simulink model "HYV_EMR_IBC_Macro_2022a"  (R2022a)
settings: Solver=ode45  StartTime=SIM.t_min  StopTime=SIM.t_simul  FixedStep=1e-2  MaxStep=10e-3  RelTol=1e-3  EnableMultiTasking=on
InitFcn:
  | init_hyv
undefined symbols (not defined in the file or in its folder): BATp, CHAp, CYCL, EDp, EMp, ICE, MTp, Paux, RDp, REDR, RegV
libraries: simulink x2
settings Model: ExtModeTrigMode=oneshot  ExtModeArmWhenConnect=off  Creator=Tony  LastModifiedBy=philippe.barrade
settings SolverCC: ZeroCrossAlgorithm=Non-adaptive  AlgebraicLoopSolver=TrustRegion
settings DataIOCC: SaveFormat=Array  SignalLoggingSaveFormat=ModelDataLogs  ReturnWorkspaceOutputs=off  SignalLoggingName=sigsOut
settings OptimizationCC: BooleanDataType=off  ExpressionDepthLimit=2147483647  LifeSpan=inf
settings DebuggingCC: SaveWithParameterizedLinksMsg=none  UnderspecifiedInitializationDetection=Classic  MergeDetectMultiDrivingBlocksExec=none  SignalResolutionControl=TryResolveAllWithWarning  MultiTaskDSMMsg=warning  MultiTaskCondExecSysMsg=none  FcnCallInpInsideContextMsg=warning  UnconnectedInputMsg=warning  UnconnectedOutputMsg=warning  UnconnectedLineMsg=warning  StateNameClashWarn=warning  SFUnexpectedBacktrackingDiag=warning  SFNoUnconditionalDefaultTransitionDiag=warning  ArithmeticOperatorsInVariantConditions=warning
settings HardwareCC: ProdBitPerPointer=32  ProdBitPerSizeT=32  ProdBitPerPtrDiffT=32  ProdLargestAtomicFloat=None  ProdIntDivRoundTo=Undefined  ProdEndianess=Unspecified  ProdWordSize=32  ProdHWDeviceType=32-bit Generic  TargetUnknown=on
settings ModelReferenceCC: PropagateSignalLabelsOutOfModel=off
settings SFSimCC: CustomCodeUndefinedFunction=UseInterfaceOnly
settings CodeAppCC: StateflowObjectComments=on
settings GRTTargetCC: TargetLangStandard=C89/C90 (ANSI)  CombineOutputUpdateFcns=off  GRTInterface=on
settings ConfigComp: CovMetricSettings=dw  CovSaveCumulativeToWorkspaceVar=on  CovSaveSingleToWorkspaceVar=on

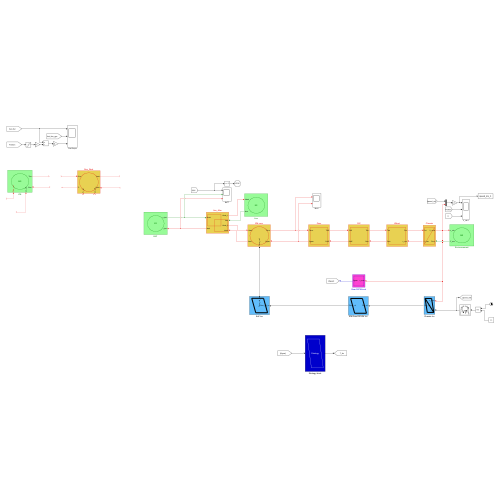
[thumbnail: Simulink's stored preview of the top-level diagram]
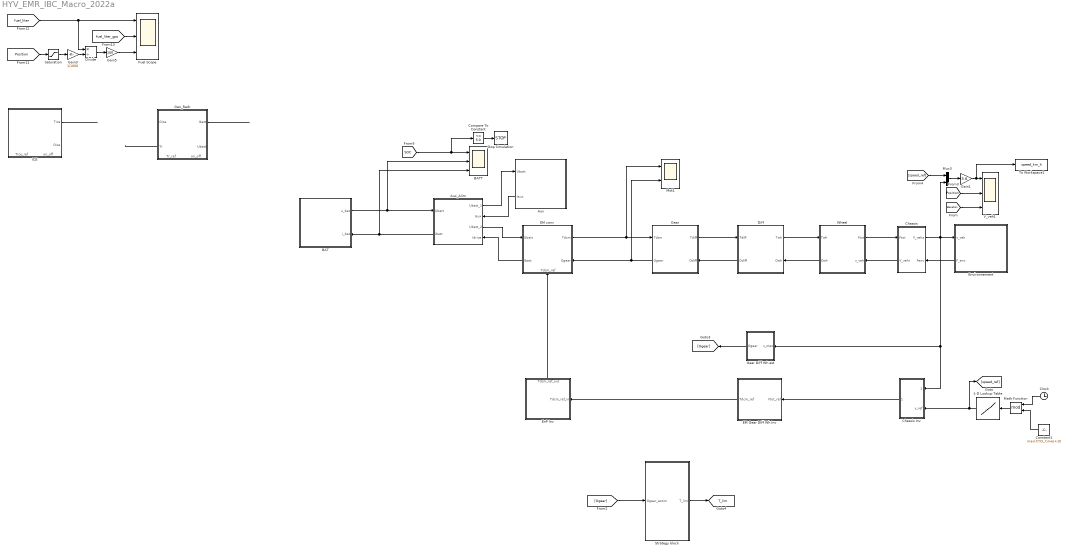
== system HYV_EMR_IBC_Macro_2022a ==
  1-D Lookup Table : Lookup_n-D  NumberOfTableDimensions=1  BreakpointsForDimension1=CYCL.time  Table=CYCL.speed  InternalRulePriority=Speed  RndMeth=Simplest
  Aux : Subsystem
      settings: PortSchema="{\"entries\":[{\"content\":{\"sides\":[{\"content\":{\"connectorIds\":[\"In1\",\"Out1\"]},\"type\":\"ConnectorPlacement.EquallySpacedRectSide\",\"uuid\":\"e57ce769-5dfa-4323-9199-18ff4bf0cf0d\"},{\"content\":{\"side\":\"RIGHT\"},\"type\":\"ConnectorPlacement.EquallySpacedRectSide\",\"uuid\":\"ab409fab-d314-4206-bddf-ed026c86ef76\"},{\"content\":{\"side\":\"TOP\"},\"type\":\"ConnectorPlacement.EquallySpacedRectSide\",\"uuid\":\"b908e240-8ad5-4078-8f5b-5b2bce20148c\"}]},\"type\":\"ConnectorPlacement.EquallySpacedConnector\",\"uuid\":\"97ae4631-eb25-4761-beab-92c01239a3fc\"}],\"packageUris\":[\"http://schema.mathworks.com/mf0/Connector/R2020b\"],\"version\":\"1.0\"}"
      mask Display:
      | plot(0,0,100,100, 1.2*[50,57.68,60.77,63.08,64.97,66.58,68,69.26,70.4, 	71.42,72.36,78.28,80,78.28,72.36,71.42,70.4, 	69.26,68,66.58,64.97,63.08,60.77,57.68,50,42.32, 	39.23,36.92,35.03,33.42,32,30.74,29.6,28.58, 	27.64,21.72,20,21.72,27.64,28.58,29.6,30.74,32, 	33.42,35.03,36.92,39.23,42.32,50]-10, 1.2*[20,21,22,23,24,25,26,27,28,29,30,40,50,60,70,71,72, 	73,74,75,76,77,78,79,80,79,78,77,76,75,74,73,72, 	71,70,60,50,40,30,29,28,27,26,25,24,23,22,21,20]-10)
      | disp('ES')
  Aux_Alim : Subsystem  mask(CM){}
      settings: PortSchema="{\"entries\":[{\"content\":{\"sides\":[{\"content\":{\"connectorIds\":[\"In1\",\"Out3\"]},\"type\":\"ConnectorPlacement.EquallySpacedRectSide\",\"uuid\":\"fe3b80e5-6bea-4454-b396-78d68e4e0983\"},{\"content\":{\"connectorIds\":[\"Out1\",\"In2\",\"Out2\",\"In3\"],\"side\":\"RIGHT\"},\"type\":\"ConnectorPlacement.EquallySpacedRectSide\",\"uuid\":\"fd9b9ae6-7a3e-4ad6-b5ff-7ff0e231c6c1\"},{\"content\":{\"side\":\"TOP\"},\"type\":\"ConnectorPlacement.EquallySpacedRectSide\",\"uuid\":\"d806e031-cf18-4ebb-a7e2-aa884fb49c19\"}]},\"type\":\"ConnectorPlacement.EquallySpacedConnector\",\"uuid\":\"fbb11b08-f3d2-4dd1-a8d6-045eff655811\"}],\"packageUris\":[\"http://schema.mathworks.com/mf0/Connector/R2020b\"],\"version\":\"1.0\"}"
      mask Display: plot(0,0,100,100,[35,35,95,95,35],[65,10,10,65,65], [5,5,65,65,5],[90,35,35,90,90])
  BAT : Subsystem
      settings: PortSchema="{\"entries\":[{\"content\":{\"sides\":[{\"content\":{\"connectorIds\":[]},\"type\":\"ConnectorPlacement.EquallySpacedRectSide\",\"uuid\":\"f966fbbf-87fd-4eae-ac75-d366ea856ba9\"},{\"content\":{\"connectorIds\":[\"Out1\",\"In1\"],\"side\":\"RIGHT\"},\"type\":\"ConnectorPlacement.EquallySpacedRectSide\",\"uuid\":\"019a522f-a65b-4de4-928a-6ec503aa07e1\"},{\"content\":{\"connectorIds\":[],\"side\":\"TOP\"},\"type\":\"ConnectorPlacement.EquallySpacedRectSide\",\"uuid\":\"2e7350c2-17d6-436e-acd0-d7bc7ebcdc21\"}]},\"type\":\"ConnectorPlacement.EquallySpacedConnector\",\"uuid\":\"cf36ffa8-c853-4b91-8b40-e4ddcf06bdb1\"}],\"packageUris\":[\"http://schema.mathworks.com/mf0/Connector/R2020b\"],\"version\":\"1.0\"}"
      mask Display:
      | plot(0,0,100,100, 1.2*[50,57.68,60.77,63.08,64.97,66.58,68,69.26,70.4, 	71.42,72.36,78.28,80,78.28,72.36,71.42,70.4, 	69.26,68,66.58,64.97,63.08,60.77,57.68,50,42.32, 	39.23,36.92,35.03,33.42,32,30.74,29.6,28.58, 	27.64,21.72,20,21.72,27.64,28.58,29.6,30.74,32, 	33.42,35.03,36.92,39.23,42.32,50]-10, 1.2*[20,21,22,23,24,25,26,27,28,29,30,40,50,60,70,71,72, 	73,74,75,76,77,78,79,80,79,78,77,76,75,74,73,72, 	71,70,60,50,40,30,29,28,27,26,25,24,23,22,21,20]-10)
      | disp('ES')
  BATT : Scope  NumInputPorts=3
  Chassis : Subsystem  mask(CM){}
      settings: PortSchema="{\"entries\":[{\"content\":{\"sides\":[{\"content\":{\"connectorIds\":[\"In1\",\"Out2\"]},\"type\":\"ConnectorPlacement.EquallySpacedRectSide\",\"uuid\":\"620ffb90-6f06-474c-af56-4865758ad724\"},{\"content\":{\"connectorIds\":[\"Out1\",\"In2\"],\"side\":\"RIGHT\"},\"type\":\"ConnectorPlacement.EquallySpacedRectSide\",\"uuid\":\"7a4bba18-9bee-4c5d-b60c-6ae6fbfa3157\"},{\"content\":{\"connectorIds\":[],\"side\":\"TOP\"},\"type\":\"ConnectorPlacement.EquallySpacedRectSide\",\"uuid\":\"2f500b5d-e16a-4b09-8380-9fc4853d3c00\"}]},\"type\":\"ConnectorPlacement.EquallySpacedConnector\",\"uuid\":\"25a91873-aa5a-4f00-84d2-bf925e985f7d\"}],\"packageUris\":[\"http://schema.mathworks.com/mf0/Connector/R2020b\"],\"version\":\"1.0\"}"
      mask Display: plot(0,0,100,100,[10,10,90,90,10],[90,10,10,90,90], [10,90],[10,90])
  Chassis Inv : Subsystem
      mask Display: plot(0,0,100,100, [10,30,90,70,10,90],[90,10,10,90,90,10])
  Clock : Clock
  Compare To Constant : simulink/Logic and Bit Operations/Compare To Constant  relop=<=  const=5.0  OutDataTypeStr=boolean
  Constant1 : Constant  Value=max(CYCL.time)+10
  Diff : Subsystem  mask(Hacheur){}
      settings: PortSchema="{\"entries\":[{\"content\":{\"sides\":[{\"content\":{\"connectorIds\":[\"In1\",\"Out2\"]},\"type\":\"ConnectorPlacement.EquallySpacedRectSide\",\"uuid\":\"61fbc010-38ff-4a80-98f4-f5d8a9e77fd8\"},{\"content\":{\"connectorIds\":[\"Out1\",\"In2\"],\"side\":\"RIGHT\"},\"type\":\"ConnectorPlacement.EquallySpacedRectSide\",\"uuid\":\"7ae9e15d-ee0f-4ba6-b3b7-5dcbca441e0a\"},{\"content\":{\"connectorIds\":[],\"side\":\"TOP\"},\"type\":\"ConnectorPlacement.EquallySpacedRectSide\",\"uuid\":\"f4fbe656-3ef3-486e-b25e-f340040f3905\"},{\"content\":{\"connectorIds\":[],\"side\":\"BOTTOM\"},\"type\":\"ConnectorPlacement.EquallySpacedRectSide\",\"uuid\":\"e8cc994c-4958-42b4-b139-c82ce4c5ea4a\"}]},\"type\":\"ConnectorPlacement.EquallySpacedConnector\",\"uuid\":\"024d92c1-e2c4-4b69-9482-c403c9d240aa\"}],\"packageUris\":[\"http://schema.mathworks.com/mf0/Connector/R2020b\"],\"version\":\"1.0\"}"
      mask Display: plot(0,0,100,100,[10,10,90,90,10],[90,10,10,90,90])
  Divide : Product  Inputs=*/
  EM Gear DIff Wh Inv : Subsystem
      mask Display: plot(0,0,100,100,[10,30,90,70,10],[90,10,10,90,90])
  EM conv : Subsystem
      settings: PortSchema="{\"entries\":[{\"content\":{\"sides\":[{\"content\":{\"connectorIds\":[\"In1\",\"Out2\"]},\"type\":\"ConnectorPlacement.EquallySpacedRectSide\",\"uuid\":\"aa766bd2-1e00-44a9-a500-41c2a98848e3\"},{\"content\":{\"connectorIds\":[\"Out1\",\"In3\"],\"side\":\"RIGHT\"},\"type\":\"ConnectorPlacement.EquallySpacedRectSide\",\"uuid\":\"49bb6889-ad6c-456e-94dd-aff29c8ca84c\"},{\"content\":{\"side\":\"TOP\"},\"type\":\"ConnectorPlacement.EquallySpacedRectSide\",\"uuid\":\"33b42b41-d96e-4f45-af15-b9a879923102\"},{\"content\":{\"connectorIds\":[\"In2\"],\"side\":\"BOTTOM\"},\"type\":\"ConnectorPlacement.EquallySpacedRectSide\",\"uuid\":\"830b03b5-14ae-4cee-8c80-baeec75b28b0\"}]},\"type\":\"ConnectorPlacement.EquallySpacedConnector\",\"uuid\":\"59a0cd24-e9fa-4621-b3e9-3869a068d1ef\"}],\"packageUris\":[\"http://schema.mathworks.com/mf0/Connector/R2020b\"],\"version\":\"1.0\"}"
      mask Display: plot(0,0,100,100, 1.4*[50,57.68,60.77,63.08,64.97,66.58,68,69.26,70.4, 	71.42,72.36,78.28,80,78.28,72.36,71.42,70.4, 	69.26,68,66.58,64.97,63.08,60.77,57.68,50,42.32, 	39.23,36.92,35.03,33.42,32,30.74,29.6,28.58, 	27.64,21.72,20,21.72,27.64,28.58,29.6,30.74,32, 	33.42,35.03,36.92,39.23,42.32,50]-20, 1.4*[20,21,22,23,24,25,26,27,28,29,30,40,50,60,70,71,72, 	73,74,75,76,77,78,79,80,79,78,77,76,75,74,73,72, 	71,70,60,50,40,30,29,28,27,26,25,24,23,22,21,20]-20)
  EnP Inv : Subsystem
      settings: PortSchema="{\"entries\":[{\"content\":{\"sides\":[{\"content\":{\"connectorIds\":[\"In1\"]},\"type\":\"ConnectorPlacement.EquallySpacedRectSide\",\"uuid\":\"39dcb6ca-7d3c-49e9-8aff-6e45c752a7e4\"},{\"content\":{\"side\":\"RIGHT\"},\"type\":\"ConnectorPlacement.EquallySpacedRectSide\",\"uuid\":\"f02eeddd-07d1-428e-b420-27aa15bc8886\"},{\"content\":{\"connectorIds\":[\"Out1\"],\"side\":\"TOP\"},\"type\":\"ConnectorPlacement.EquallySpacedRectSide\",\"uuid\":\"752f1347-9d6b-4136-bea0-6d91d7e60b0a\"}]},\"type\":\"ConnectorPlacement.EquallySpacedConnector\",\"uuid\":\"f213fa59-4ba1-490d-8e30-b1e1c9b24a7e\"}],\"packageUris\":[\"http://schema.mathworks.com/mf0/Connector/R2020b\"],\"version\":\"1.0\"}"
      mask Display: plot(0,0,100,100,[10,30,90,70,10],[90,10,10,90,90])
  Environnement : Subsystem
      settings: PortSchema="{\"entries\":[{\"content\":{\"sides\":[{\"content\":{\"connectorIds\":[\"In1\",\"Out1\"]},\"type\":\"ConnectorPlacement.EquallySpacedRectSide\",\"uuid\":\"f966fbbf-87fd-4eae-ac75-d366ea856ba9\"},{\"content\":{\"connectorIds\":[],\"side\":\"RIGHT\"},\"type\":\"ConnectorPlacement.EquallySpacedRectSide\",\"uuid\":\"019a522f-a65b-4de4-928a-6ec503aa07e1\"},{\"content\":{\"connectorIds\":[],\"side\":\"TOP\"},\"type\":\"ConnectorPlacement.EquallySpacedRectSide\",\"uuid\":\"2e7350c2-17d6-436e-acd0-d7bc7ebcdc21\"}]},\"type\":\"ConnectorPlacement.EquallySpacedConnector\",\"uuid\":\"cf36ffa8-c853-4b91-8b40-e4ddcf06bdb1\"}],\"packageUris\":[\"http://schema.mathworks.com/mf0/Connector/R2020b\"],\"version\":\"1.0\"}"
      mask Display:
      | plot(0,0,100,100, 1.2*[50,57.68,60.77,63.08,64.97,66.58,68,69.26,70.4, 	71.42,72.36,78.28,80,78.28,72.36,71.42,70.4, 	69.26,68,66.58,64.97,63.08,60.77,57.68,50,42.32, 	39.23,36.92,35.03,33.42,32,30.74,29.6,28.58, 	27.64,21.72,20,21.72,27.64,28.58,29.6,30.74,32, 	33.42,35.03,36.92,39.23,42.32,50]-10, 1.2*[20,21,22,23,24,25,26,27,28,29,30,40,50,60,70,71,72, 	73,74,75,76,77,78,79,80,79,78,77,76,75,74,73,72, 	71,70,60,50,40,30,29,28,27,26,25,24,23,22,21,20]-10)
      | disp('MS')
  Fuel Scope : Scope  NumInputPorts=3
  Gain1 : Gain  Gain=3.6
  Gain3 : Gain  Gain=1/1000
  Gain5 : Gain  Gain=100
  Gear : Subsystem  mask(Hacheur){}
      settings: PortSchema="{\"entries\":[{\"content\":{\"sides\":[{\"content\":{\"connectorIds\":[\"In1\",\"Out2\"]},\"type\":\"ConnectorPlacement.EquallySpacedRectSide\",\"uuid\":\"61fbc010-38ff-4a80-98f4-f5d8a9e77fd8\"},{\"content\":{\"connectorIds\":[\"Out1\",\"In2\"],\"side\":\"RIGHT\"},\"type\":\"ConnectorPlacement.EquallySpacedRectSide\",\"uuid\":\"7ae9e15d-ee0f-4ba6-b3b7-5dcbca441e0a\"},{\"content\":{\"connectorIds\":[],\"side\":\"TOP\"},\"type\":\"ConnectorPlacement.EquallySpacedRectSide\",\"uuid\":\"f4fbe656-3ef3-486e-b25e-f340040f3905\"},{\"content\":{\"connectorIds\":[],\"side\":\"BOTTOM\"},\"type\":\"ConnectorPlacement.EquallySpacedRectSide\",\"uuid\":\"e8cc994c-4958-42b4-b139-c82ce4c5ea4a\"}]},\"type\":\"ConnectorPlacement.EquallySpacedConnector\",\"uuid\":\"024d92c1-e2c4-4b69-9482-c403c9d240aa\"}],\"packageUris\":[\"http://schema.mathworks.com/mf0/Connector/R2020b\"],\"version\":\"1.0\"}"
      mask Display: plot(0,0,100,100,[10,10,90,90,10],[90,10,10,90,90])
  Gear Diff Wh est : Subsystem  mask(Hacheur){}
      settings: PortSchema="{\"entries\":[{\"content\":{\"sides\":[{\"content\":{\"connectorIds\":[\"Out1\"]},\"type\":\"ConnectorPlacement.EquallySpacedRectSide\",\"uuid\":\"97b10c34-40f1-482d-a289-d09ab630d3a5\"},{\"content\":{\"connectorIds\":[\"In1\"],\"side\":\"RIGHT\"},\"type\":\"ConnectorPlacement.EquallySpacedRectSide\",\"uuid\":\"48711657-cfab-4e40-bd05-7e981abf95c6\"},{\"content\":{\"connectorIds\":[],\"side\":\"TOP\"},\"type\":\"ConnectorPlacement.EquallySpacedRectSide\",\"uuid\":\"ae2d6315-1874-4483-90e6-e233be87d834\"}]},\"type\":\"ConnectorPlacement.EquallySpacedConnector\",\"uuid\":\"72cd56a5-d150-4d8c-8f1b-f53960fc3550\"}],\"packageUris\":[\"http://schema.mathworks.com/mf0/Connector/R2020b\"],\"version\":\"1.0\"}"
      mask Display: plot(0,0,100,100,[10,10,90,90,10],[90,10,10,90,90])
  Gen_Redr : Subsystem
      settings: PortSchema="{\"entries\":[{\"content\":{\"sides\":[{\"content\":{\"connectorIds\":[\"In1\",\"Out2\"]},\"type\":\"ConnectorPlacement.EquallySpacedRectSide\",\"uuid\":\"aa766bd2-1e00-44a9-a500-41c2a98848e3\"},{\"content\":{\"connectorIds\":[\"Out1\",\"In4\"],\"side\":\"RIGHT\"},\"type\":\"ConnectorPlacement.EquallySpacedRectSide\",\"uuid\":\"49bb6889-ad6c-456e-94dd-aff29c8ca84c\"},{\"content\":{\"side\":\"TOP\"},\"type\":\"ConnectorPlacement.EquallySpacedRectSide\",\"uuid\":\"33b42b41-d96e-4f45-af15-b9a879923102\"},{\"content\":{\"connectorIds\":[\"In2\",\"In3\"],\"side\":\"BOTTOM\"},\"type\":\"ConnectorPlacement.EquallySpacedRectSide\",\"uuid\":\"830b03b5-14ae-4cee-8c80-baeec75b28b0\"}]},\"type\":\"ConnectorPlacement.EquallySpacedConnector\",\"uuid\":\"59a0cd24-e9fa-4621-b3e9-3869a068d1ef\"}],\"packageUris\":[\"http://schema.mathworks.com/mf0/Connector/R2020b\"],\"version\":\"1.0\"}"
      mask Display: plot(0,0,100,100, 1.4*[50,57.68,60.77,63.08,64.97,66.58,68,69.26,70.4, 	71.42,72.36,78.28,80,78.28,72.36,71.42,70.4, 	69.26,68,66.58,64.97,63.08,60.77,57.68,50,42.32, 	39.23,36.92,35.03,33.42,32,30.74,29.6,28.58, 	27.64,21.72,20,21.72,27.64,28.58,29.6,30.74,32, 	33.42,35.03,36.92,39.23,42.32,50]-20, 1.4*[20,21,22,23,24,25,26,27,28,29,30,40,50,60,70,71,72, 	73,74,75,76,77,78,79,80,79,78,77,76,75,74,73,72, 	71,70,60,50,40,30,29,28,27,26,25,24,23,22,21,20]-20)
  ICE : Subsystem
      settings: PortSchema="{\"entries\":[{\"content\":{\"sides\":[{\"content\":{},\"type\":\"ConnectorPlacement.EquallySpacedRectSide\",\"uuid\":\"5e0004dc-9353-4505-bdf1-6128bddb82fb\"},{\"content\":{\"connectorIds\":[\"Out1\",\"In3\"],\"side\":\"RIGHT\"},\"type\":\"ConnectorPlacement.EquallySpacedRectSide\",\"uuid\":\"6fc81608-8d8e-4e86-94d9-80743178a522\"},{\"content\":{\"side\":\"TOP\"},\"type\":\"ConnectorPlacement.EquallySpacedRectSide\",\"uuid\":\"4904ac3e-9806-48bd-b6d0-39ab169c5dfc\"},{\"content\":{\"connectorIds\":[\"In1\",\"In2\"],\"side\":\"BOTTOM\"},\"type\":\"ConnectorPlacement.EquallySpacedRectSide\",\"uuid\":\"82cbcfdd-da9c-4107-ad22-b08b0e6750b1\"}]},\"type\":\"ConnectorPlacement.EquallySpacedConnector\",\"uuid\":\"e4ba4c66-9db2-4dbc-8ef6-8857e646fcbd\"}],\"packageUris\":[\"http://schema.mathworks.com/mf0/Connector/R2020b\"],\"version\":\"1.0\"}"
      mask Display:
      | plot(0,0,100,100, 1.2*[50,57.68,60.77,63.08,64.97,66.58,68,69.26,70.4, 	71.42,72.36,78.28,80,78.28,72.36,71.42,70.4, 	69.26,68,66.58,64.97,63.08,60.77,57.68,50,42.32, 	39.23,36.92,35.03,33.42,32,30.74,29.6,28.58, 	27.64,21.72,20,21.72,27.64,28.58,29.6,30.74,32, 	33.42,35.03,36.92,39.23,42.32,50]-10, 1.2*[20,21,22,23,24,25,26,27,28,29,30,40,50,60,70,71,72, 	73,74,75,76,77,78,79,80,79,78,77,76,75,74,73,72, 	71,70,60,50,40,30,29,28,27,26,25,24,23,22,21,20]-10)
      | disp('MS')
  Math Function : Math  Operator=mod
  Mot1 : Scope  NumInputPorts=2
  Mux3 : Mux  Inputs=2
  Saturation : Saturate  UpperLimit=inf  LowerLimit=10.0
  Stop Simulation : Stop
  Strategy block : Subsystem
      settings: PortSchema="{\"entries\":[{\"content\":{\"sides\":[{\"content\":{\"connectorIds\":[\"Out1\"]},\"type\":\"ConnectorPlacement.EquallySpacedRectSide\",\"uuid\":\"4c676ab4-47cc-4f87-ad93-ce3a4db5a06a\"},{\"content\":{\"connectorIds\":[\"In1\"],\"side\":\"RIGHT\"},\"type\":\"ConnectorPlacement.EquallySpacedRectSide\",\"uuid\":\"84b1a57b-73c9-4ed3-8724-d96f85b248dd\"},{\"content\":{\"side\":\"TOP\"},\"type\":\"ConnectorPlacement.EquallySpacedRectSide\",\"uuid\":\"73aa9894-9e21-4e9a-8a0b-0eeb601767d1\"}]},\"type\":\"ConnectorPlacement.EquallySpacedConnector\",\"uuid\":\"1d658a79-37bf-4296-a4f6-ebfe26a5ed36\"}],\"packageUris\":[\"http://schema.mathworks.com/mf0/Connector/R2020b\"],\"version\":\"1.0\"}"
      mask Display:
      | color('white')
      | plot(0,0,100,100,[10,30,90,70,10],[90,10,10,90,90])
      | disp('Strategy')
  To Workspace1 : ToWorkspace  VariableName=speed_km_h  SampleTime=-1
  V_veh1 : Scope  NumInputPorts=3
  Wheel : Subsystem  mask(Hacheur){}
      settings: PortSchema="{\"entries\":[{\"content\":{\"sides\":[{\"content\":{\"connectorIds\":[\"In1\",\"Out2\"]},\"type\":\"ConnectorPlacement.EquallySpacedRectSide\",\"uuid\":\"61fbc010-38ff-4a80-98f4-f5d8a9e77fd8\"},{\"content\":{\"connectorIds\":[\"Out1\",\"In2\"],\"side\":\"RIGHT\"},\"type\":\"ConnectorPlacement.EquallySpacedRectSide\",\"uuid\":\"7ae9e15d-ee0f-4ba6-b3b7-5dcbca441e0a\"},{\"content\":{\"connectorIds\":[],\"side\":\"TOP\"},\"type\":\"ConnectorPlacement.EquallySpacedRectSide\",\"uuid\":\"f4fbe656-3ef3-486e-b25e-f340040f3905\"},{\"content\":{\"connectorIds\":[],\"side\":\"BOTTOM\"},\"type\":\"ConnectorPlacement.EquallySpacedRectSide\",\"uuid\":\"e8cc994c-4958-42b4-b139-c82ce4c5ea4a\"}]},\"type\":\"ConnectorPlacement.EquallySpacedConnector\",\"uuid\":\"024d92c1-e2c4-4b69-9482-c403c9d240aa\"}],\"packageUris\":[\"http://schema.mathworks.com/mf0/Connector/R2020b\"],\"version\":\"1.0\"}"
      mask Display: plot(0,0,100,100,[10,10,90,90,10],[90,10,10,90,90])
  tag scope: T_lim=global
  wires:
  [SOC] -> Compare To Constant/1, BATT/1
  Compare To Constant/1 -> Stop Simulation/1
  Gear/2(Ogear) -> EM conv/3(Ogear), Mot1/2
  EM conv/1(Tdcm) -> Mot1/1, Gear/1(Tdcm)
  Wheel/1(Ftot) -> Chassis/1(Ftot)
  Wheel/2(Owh) -> Diff/2(Owh)
  Chassis/2(V_vehr) -> Wheel/2(v_veh)
  Diff/2(Odiff) -> Gear/2(Odiff)
  Diff/1(Twh) -> Wheel/1(Twh)
  Gear/1(Tdiff) -> Diff/1(Tdiff)
  Environnement/1(F_env) -> Chassis/2(Fenv)
  EM Gear DIff Wh Inv/1(Tdcm_ref) -> EnP Inv/1(Tdcm_ref_in)
  Chassis Inv/1(Ftot_ref) -> EM Gear DIff Wh Inv/1(Ftot_ref)
  1-D Lookup Table/1 -> Chassis Inv/2(v_ref), [speed_ref]
  [Ogear] -> Strategy block/1(Ogear_estim)
  Gear Diff Wh est/1(Ogear) -> [Ogear]
  Strategy block/1(T_lim) -> [T_lim]
  Mux3/1 -> Gain1/1
  [Elevation] -> V_veh1/3
  [speed_ref] -> Mux3/1
  [Position] -> V_veh1/2
  Gain1/1 -> To Workspace1/1, V_veh1/1
  Chassis/1(V_veha) -> Mux3/2, Gear Diff Wh est/1(v_mes), Chassis Inv/1(v_mes), Environnement/1(v_veh)
  EnP Inv/1(Tdcm_ref_out) -> EM conv/2(Tdcm_ref)
  Divide/1 -> Gain5/1
  Gain3/1 -> Divide/2
  [fuel_liter_gps] -> Fuel Scope/2
  [Position] -> Saturation/1
  Gain5/1 -> Fuel Scope/3
  [fuel_liter] -> Fuel Scope/1, Divide/1
  Saturation/1 -> Gain3/1
  ICE/1(Tice) -> ?
  ? -> ICE/3(Oice)
  ? -> Gen_Redr/1(Oice)
  Gen_Redr/2(Tr) -> ?
  ? -> Gen_Redr/4(Ubatt)
  Gen_Redr/1(Ibatt) -> ?
  Aux_Alim/2(Ubatt_2) -> EM conv/1(Ubatt)
  EM conv/2(Ibatt) -> Aux_Alim/3(Idrive)
  Aux_Alim/1(Ubatt_1) -> Aux/1(Ubatt)
  Aux/1(Iaux) -> Aux_Alim/2(Iaux)
  Aux_Alim/3(Ibatt) -> BATT/3, BAT/1(i_bat)
  BAT/1(u_bat) -> BATT/2, Aux_Alim/1(Ubatt)
  Math Function/1 -> 1-D Lookup Table/1
  Clock/1 -> Math Function/1
  Constant1/1 -> Math Function/2
  ? -> ICE/1(Tice_ref)
  ? -> ICE/2(on_off)

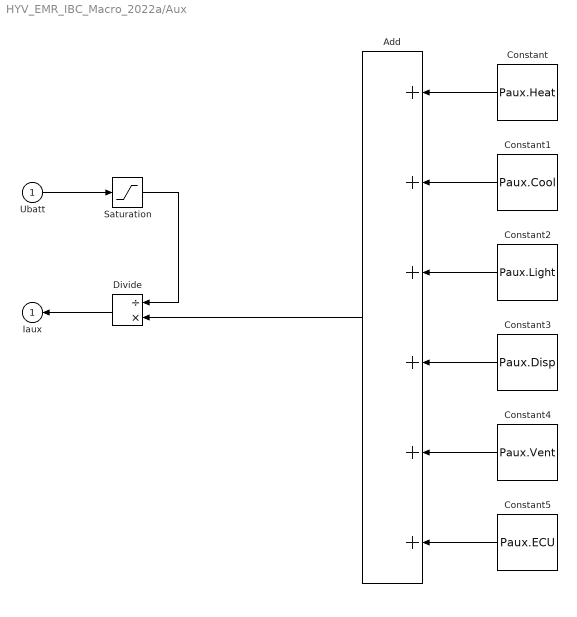
== system HYV_EMR_IBC_Macro_2022a/Aux ==
  Ubatt : Inport
  Add : Sum  Inputs=++++++
  Constant : Constant  Value=Paux.Heat
  Constant1 : Constant  Value=Paux.Cool
  Constant2 : Constant  Value=Paux.Light
  Constant3 : Constant  Value=Paux.Disp
  Constant4 : Constant  Value=Paux.Vent
  Constant5 : Constant  Value=Paux.ECU
  Divide : Product  Inputs=/*
  Saturation : Saturate  UpperLimit=inf  LowerLimit=10.0
  Iaux : Outport  InitialOutput=0
  wires:
  Constant2/1 -> Add/3
  Constant1/1 -> Add/2
  Constant/1 -> Add/1
  Constant3/1 -> Add/4
  Constant4/1 -> Add/5
  Constant5/1 -> Add/6
  Ubatt/1 -> Saturation/1
  Divide/1 -> Iaux/1
  Saturation/1 -> Divide/1
  Add/1 -> Divide/2

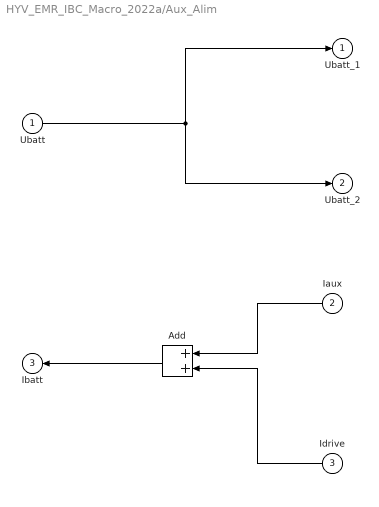
== system HYV_EMR_IBC_Macro_2022a/Aux_Alim ==
  Ubatt : Inport
  Iaux : Inport  Port=2
  Idrive : Inport  Port=3
  Add : Sum
  Ubatt_1 : Outport  InitialOutput=0
  Ubatt_2 : Outport  Port=2  InitialOutput=0
  Ibatt : Outport  Port=3  InitialOutput=0
  wires:
  Ubatt/1 -> Ubatt_2/1, Ubatt_1/1
  Iaux/1 -> Add/1
  Idrive/1 -> Add/2
  Add/1 -> Ibatt/1

== system HYV_EMR_IBC_Macro_2022a/BAT ==
  i_bat : Inport
  Adaptation : Subsystem  mask(CM){}
      settings: PortSchema="{\"entries\":[{\"content\":{\"sides\":[{\"content\":{\"connectorIds\":[\"In1\",\"Out2\"]},\"type\":\"ConnectorPlacement.EquallySpacedRectSide\",\"uuid\":\"43b53794-c784-4d35-8a91-f1490638489e\"},{\"content\":{\"connectorIds\":[\"Out1\",\"In2\"],\"side\":\"RIGHT\"},\"type\":\"ConnectorPlacement.EquallySpacedRectSide\",\"uuid\":\"00b1a1a6-7269-4083-abb9-f1208d9f3b4c\"},{\"content\":{\"connectorIds\":[],\"side\":\"TOP\"},\"type\":\"ConnectorPlacement.EquallySpacedRectSide\",\"uuid\":\"3919f87a-9a68-4334-b84e-5fe8c9917a96\"}]},\"type\":\"ConnectorPlacement.EquallySpacedConnector\",\"uuid\":\"9597a696-d499-48cc-bc44-63d792d74754\"}],\"packageUris\":[\"http://schema.mathworks.com/mf0/Connector/R2020b\"],\"version\":\"1.0\"}"
      mask Display: plot(0,0,100,100, [10,10,90,90,10],[90,10,10,90,90], [90,10,90],[10,50,90])
  Battery  cell resistance : Subsystem  mask(Hacheur){}
      settings: PortSchema="{\"entries\":[{\"content\":{\"sides\":[{\"content\":{\"connectorIds\":[\"In1\",\"Out2\"]},\"type\":\"ConnectorPlacement.EquallySpacedRectSide\",\"uuid\":\"43b53794-c784-4d35-8a91-f1490638489e\"},{\"content\":{\"connectorIds\":[\"Out1\",\"In2\"],\"side\":\"RIGHT\"},\"type\":\"ConnectorPlacement.EquallySpacedRectSide\",\"uuid\":\"00b1a1a6-7269-4083-abb9-f1208d9f3b4c\"},{\"content\":{\"connectorIds\":[],\"side\":\"TOP\"},\"type\":\"ConnectorPlacement.EquallySpacedRectSide\",\"uuid\":\"3919f87a-9a68-4334-b84e-5fe8c9917a96\"}]},\"type\":\"ConnectorPlacement.EquallySpacedConnector\",\"uuid\":\"9597a696-d499-48cc-bc44-63d792d74754\"}],\"packageUris\":[\"http://schema.mathworks.com/mf0/Connector/R2020b\"],\"version\":\"1.0\"}"
      mask Display: plot(0,0,100,100,[10,10,90,90,10],[90,10,10,90,90])
  OCV Source : Subsystem
      settings: PortSchema="{\"entries\":[{\"content\":{\"sides\":[{\"content\":{\"connectorIds\":[]},\"type\":\"ConnectorPlacement.EquallySpacedRectSide\",\"uuid\":\"87b7c904-bcc3-4a98-87e1-6b58a76e8897\"},{\"content\":{\"connectorIds\":[\"Out1\",\"In1\"],\"side\":\"RIGHT\"},\"type\":\"ConnectorPlacement.EquallySpacedRectSide\",\"uuid\":\"67c0e4e9-ec6a-4f26-b099-e0fb0eaa0b35\"},{\"content\":{\"connectorIds\":[],\"side\":\"TOP\"},\"type\":\"ConnectorPlacement.EquallySpacedRectSide\",\"uuid\":\"8fb5181e-f6b7-4828-b0d6-b00809980f9d\"}]},\"type\":\"ConnectorPlacement.EquallySpacedConnector\",\"uuid\":\"ac4387ff-8ed1-4b4c-b503-b7c8237b5a9a\"}],\"packageUris\":[\"http://schema.mathworks.com/mf0/Connector/R2020b\"],\"version\":\"1.0\"}"
      mask Display:
      | plot(0,0,100,100, 1.2*[50,57.68,60.77,63.08,64.97,66.58,68,69.26,70.4, 	71.42,72.36,78.28,80,78.28,72.36,71.42,70.4, 	69.26,68,66.58,64.97,63.08,60.77,57.68,50,42.32, 	39.23,36.92,35.03,33.42,32,30.74,29.6,28.58, 	27.64,21.72,20,21.72,27.64,28.58,29.6,30.74,32, 	33.42,35.03,36.92,39.23,42.32,50]-10, 1.2*[20,21,22,23,24,25,26,27,28,29,30,40,50,60,70,71,72, 	73,74,75,76,77,78,79,80,79,78,77,76,75,74,73,72, 	71,70,60,50,40,30,29,28,27,26,25,24,23,22,21,20]-10)
      | disp('MS')
  u_bat : Outport  InitialOutput=0
  wires:
  Adaptation/1(u_bat) -> u_bat/1
  i_bat/1 -> Adaptation/2(I_bat)
  Adaptation/2(i_cell) -> Battery  cell resistance/2(icell)
  Battery  cell resistance/1(u_cell) -> Adaptation/1(u_cell)
  OCV Source/1(OCV) -> Battery  cell resistance/1(OCV)
  Battery  cell resistance/2(I_cell) -> OCV Source/1("I_cell ")

== system HYV_EMR_IBC_Macro_2022a/Chassis ==
  Ftot : Inport
  Fenv : Inport  Port=2
  Add : Sum  Inputs=+-
  Gain : Gain  Gain=1/(CHAp.M_eq+EMp.J*(MTp.k_gear*MTp.k_diff/MTp.R_wheel)^2)
  Integrator : Integrator
  V_veha : Outport  InitialOutput=0
  V_vehr : Outport  Port=2  InitialOutput=0
  wires:
  Ftot/1 -> Add/1
  Add/1 -> Gain/1
  Gain/1 -> Integrator/1
  Integrator/1 -> V_veha/1, V_vehr/1
  Fenv/1 -> Add/2

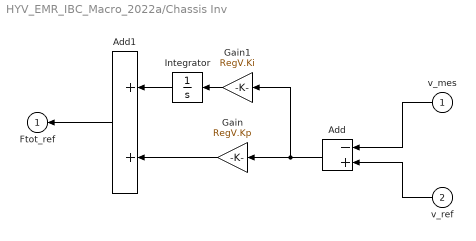
== system HYV_EMR_IBC_Macro_2022a/Chassis Inv ==
  v_mes : Inport
  v_ref : Inport  Port=2
  Add : Sum  Inputs=-+
  Add1 : Sum
  Gain : Gain  Gain=RegV.Kp
  Gain1 : Gain  Gain=RegV.Ki
  Integrator : Integrator
  Ftot_ref : Outport  InitialOutput=0
  wires:
  v_ref/1 -> Add/2
  v_mes/1 -> Add/1
  Add/1 -> Gain1/1, Gain/1
  Gain1/1 -> Integrator/1
  Gain/1 -> Add1/2
  Add1/1 -> Ftot_ref/1
  Integrator/1 -> Add1/1

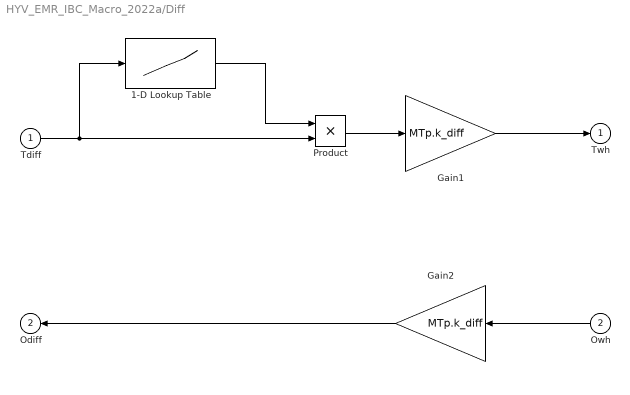
== system HYV_EMR_IBC_Macro_2022a/Diff ==
  Tdiff : Inport
  Owh : Inport  Port=2
  1-D Lookup Table : Lookup_n-D  NumberOfTableDimensions=1  BreakpointsForDimension1=[-500 -200 -10 0 10 200 500]  Table=[1/MTp.diff_eff 1/MTp.diff_eff 1/MTp.diff_eff 0 MTp.diff_eff MTp.diff_eff MTp.diff_eff]  InternalRulePriority=Speed  RndMeth=Simplest
  Gain1 : Gain  Gain=MTp.k_diff
  Gain2 : Gain  Gain=MTp.k_diff
  Product : Product
  Twh : Outport  InitialOutput=0
  Odiff : Outport  Port=2  InitialOutput=0
  wires:
  Gain1/1 -> Twh/1
  Tdiff/1 -> Product/2, 1-D Lookup Table/1
  Gain2/1 -> Odiff/1
  Owh/1 -> Gain2/1
  Product/1 -> Gain1/1
  1-D Lookup Table/1 -> Product/1

== system HYV_EMR_IBC_Macro_2022a/EM Gear DIff Wh Inv ==
  Ftot_ref : Inport
  Gain : Gain  Gain=-1
  Gain2 : Gain  Gain=1/(MTp.k_gear*MTp.k_diff/MTp.R_wheel)
  Saturation Dynamic : simulink/Discontinuities/Saturation Dynamic  OutMin=[]  OutMax=[]  OutDataTypeStr=Inherit: Same as second input  OutDataType=fixdt(1, 16)  OutScaling=2^-10  DoSatur=off
  Tdcm_ref : Outport  InitialOutput=0
  wires:
  Ftot_ref/1 -> Gain2/1
  Saturation Dynamic/1 -> Tdcm_ref/1
  Gain2/1 -> Saturation Dynamic/2
  Gain/1 -> Saturation Dynamic/3
  [T_lim] -> Gain/1, Saturation Dynamic/1

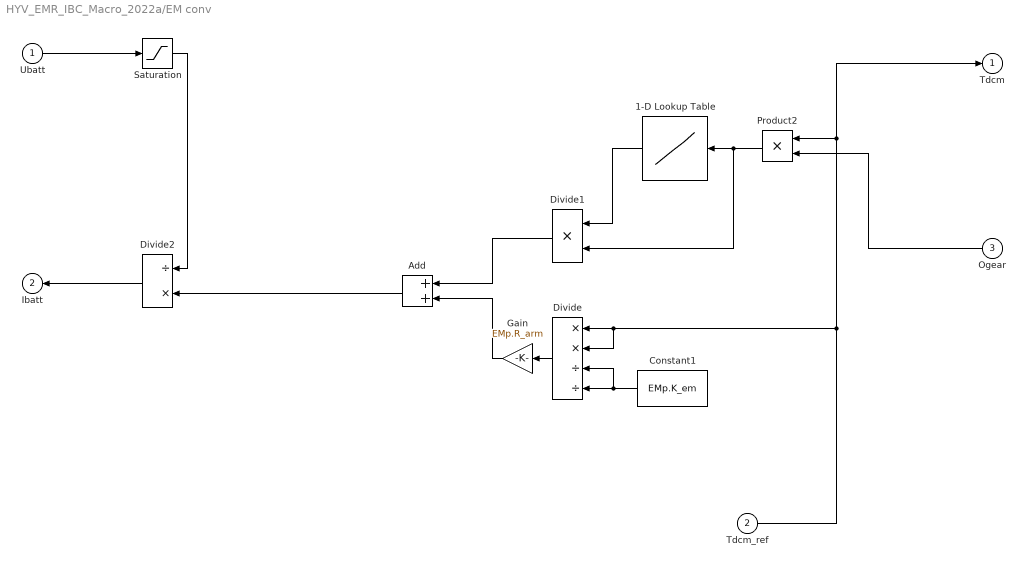
== system HYV_EMR_IBC_Macro_2022a/EM conv ==
  Ubatt : Inport
  Tdcm_ref : Inport  Port=2
  Ogear : Inport  Port=3
  1-D Lookup Table : Lookup_n-D  NumberOfTableDimensions=1  BreakpointsForDimension1=[-150e3 -10 0 10 150e3]  Table=[EDp.eff EDp.eff 1 1/EDp.eff 1/EDp.eff]  InternalRulePriority=Speed  RndMeth=Simplest
  Add : Sum
  Constant1 : Constant  Value=EMp.K_em
  Divide : Product  Inputs=**//
  Divide1 : Product  Inputs=**
  Divide2 : Product  Inputs=/*
  Gain : Gain  Gain=EMp.R_arm
  Product2 : Product
  Saturation : Saturate  UpperLimit=inf  LowerLimit=1.0
  Tdcm : Outport  InitialOutput=0
  Ibatt : Outport  Port=2  InitialOutput=0
  wires:
  Product2/1 -> Divide1/2, 1-D Lookup Table/1
  Ogear/1 -> Product2/2
  1-D Lookup Table/1 -> Divide1/1
  Tdcm_ref/1 -> Divide/2, Divide/1, Tdcm/1, Product2/1
  Constant1/1 -> Divide/3, Divide/4
  Divide1/1 -> Add/1
  Divide/1 -> Gain/1
  Ubatt/1 -> Saturation/1
  Divide2/1 -> Ibatt/1
  Add/1 -> Divide2/2
  Saturation/1 -> Divide2/1
  Gain/1 -> Add/2

== system HYV_EMR_IBC_Macro_2022a/EnP Inv ==
  Tdcm_ref_in : Inport
  Tdcm_ref_out : Outport  InitialOutput=0
  wires:
  Tdcm_ref_in/1 -> Tdcm_ref_out/1

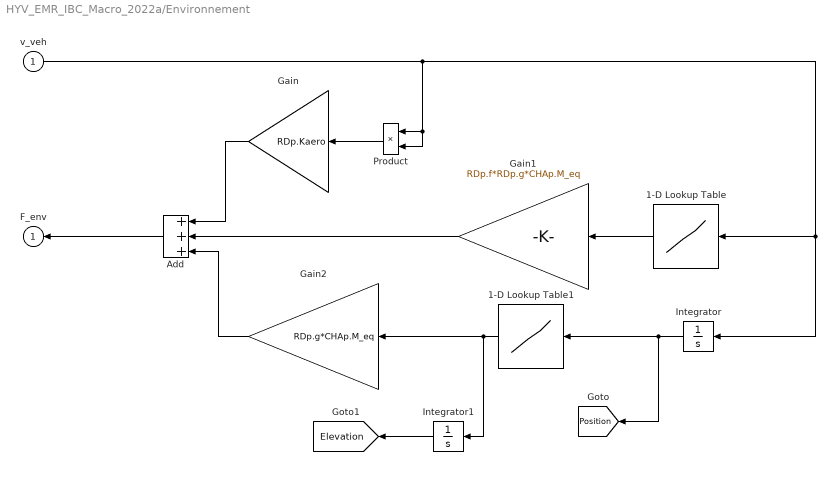
== system HYV_EMR_IBC_Macro_2022a/Environnement ==
  v_veh : Inport
  1-D Lookup Table : Lookup_n-D  NumberOfTableDimensions=1  BreakpointsForDimension1=[-100 -1 0 1 100]  Table=[-1 -1 0 1 1]  InternalRulePriority=Speed  RndMeth=Simplest
  1-D Lookup Table1 : Lookup_n-D  NumberOfTableDimensions=1  BreakpointsForDimension1=CYCL.position  Table=CYCL.slope  InternalRulePriority=Speed  RndMeth=Simplest
  Add : Sum  Inputs=+++
  Gain : Gain  Gain=RDp.Kaero  SaturateOnIntegerOverflow=on  OutDataTypeStr=Inherit: Same as input  ParamDataTypeStr=Inherit: Same as input
  Gain1 : Gain  Gain=RDp.f*RDp.g*CHAp.M_eq  SaturateOnIntegerOverflow=on  OutDataTypeStr=Inherit: Same as input  ParamDataTypeStr=Inherit: Same as input
  Gain2 : Gain  Gain=RDp.g*CHAp.M_eq  SaturateOnIntegerOverflow=on  OutDataTypeStr=Inherit: Same as input  ParamDataTypeStr=Inherit: Same as input
  Integrator : Integrator
  Integrator1 : Integrator
  Product : Product  InputSameDT=on  SaturateOnIntegerOverflow=on  OutDataTypeStr=Inherit: Same as first input
  F_env : Outport  InitialOutput=0
  tag scope: Elevation=global, Position=global
  wires:
  Product/1 -> Gain/1
  Add/1 -> F_env/1
  v_veh/1 -> Product/1, Product/2, Integrator/1, 1-D Lookup Table/1
  Gain/1 -> Add/1
  Gain1/1 -> Add/2
  1-D Lookup Table/1 -> Gain1/1
  Integrator/1 -> 1-D Lookup Table1/1, [Position]
  1-D Lookup Table1/1 -> Gain2/1, Integrator1/1
  Gain2/1 -> Add/3
  Integrator1/1 -> [Elevation]

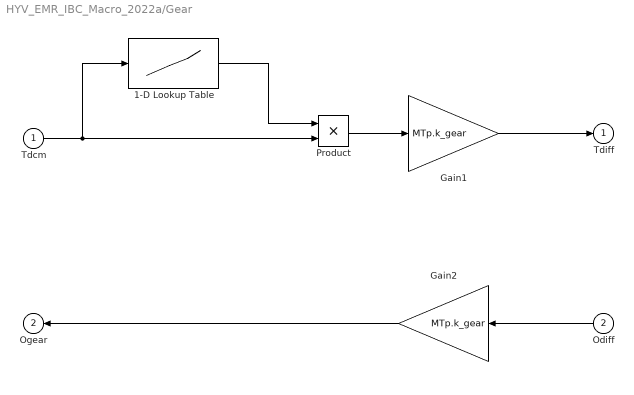
== system HYV_EMR_IBC_Macro_2022a/Gear ==
  Tdcm : Inport
  Odiff : Inport  Port=2
  1-D Lookup Table : Lookup_n-D  NumberOfTableDimensions=1  BreakpointsForDimension1=[-500 -200 -10 0 10 200 500]  Table=[1/MTp.Gear_eff 1/MTp.Gear_eff 1/MTp.Gear_eff 0 MTp.Gear_eff MTp.Gear_eff MTp.Gear_eff]  InternalRulePriority=Speed  RndMeth=Simplest
  Gain1 : Gain  Gain=MTp.k_gear
  Gain2 : Gain  Gain=MTp.k_gear
  Product : Product
  Tdiff : Outport  InitialOutput=0
  Ogear : Outport  Port=2  InitialOutput=0
  wires:
  Gain1/1 -> Tdiff/1
  Tdcm/1 -> Product/2, 1-D Lookup Table/1
  Gain2/1 -> Ogear/1
  Odiff/1 -> Gain2/1
  Product/1 -> Gain1/1
  1-D Lookup Table/1 -> Product/1

== system HYV_EMR_IBC_Macro_2022a/Gear Diff Wh est ==
  v_mes : Inport
  Gain2 : Gain  Gain=MTp.k_gear*MTp.k_diff/MTp.R_wheel
  Ogear : Outport  InitialOutput=0
  wires:
  v_mes/1 -> Gain2/1
  Gain2/1 -> Ogear/1

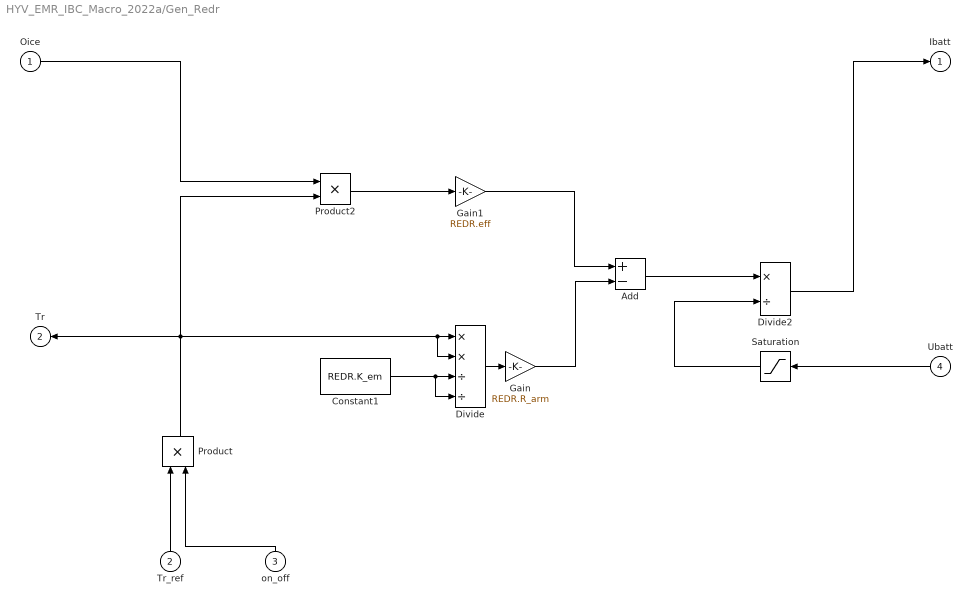
== system HYV_EMR_IBC_Macro_2022a/Gen_Redr ==
  Oice : Inport
  Tr_ref : Inport  Port=2
  on_off : Inport  Port=3
  Ubatt : Inport  Port=4
  Add : Sum  Inputs=+-
  Constant1 : Constant  Value=REDR.K_em
  Divide : Product  Inputs=**//
  Divide2 : Product  Inputs=*/
  Gain : Gain  Gain=REDR.R_arm
  Gain1 : Gain  Gain=REDR.eff
  Product : Product  RndMeth=Zero
  Product2 : Product
  Saturation : Saturate  UpperLimit=inf  LowerLimit=1.0
  Ibatt : Outport  InitialOutput=0
  Tr : Outport  Port=2  InitialOutput=0
  wires:
  Product2/1 -> Gain1/1
  Constant1/1 -> Divide/3, Divide/4
  Divide/1 -> Gain/1
  Oice/1 -> Product2/1
  Gain1/1 -> Add/1
  Gain/1 -> Add/2
  Add/1 -> Divide2/1
  Ubatt/1 -> Saturation/1
  Divide2/1 -> Ibatt/1
  Saturation/1 -> Divide2/2
  Tr_ref/1 -> Product/1
  Product/1 -> Product2/2, Tr/1, Divide/2, Divide/1
  on_off/1 -> Product/2

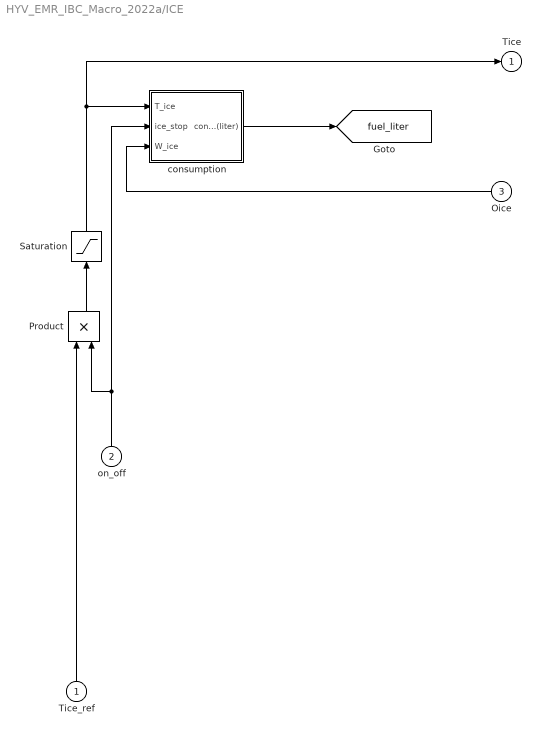
== system HYV_EMR_IBC_Macro_2022a/ICE ==
  Tice_ref : Inport
  on_off : Inport  Port=2
  Oice : Inport  Port=3
  Product : Product  RndMeth=Zero
  Saturation : Saturate  UpperLimit=102  LowerLimit=0
  consumption : Subsystem
  Tice : Outport  InitialOutput=0  VectorParamsAs1DForOutWhenUnconnected=off
  tag scope: fuel_liter=global
  wires:
  on_off/1 -> consumption/2(ice_stop), Product/2
  Product/1 -> Saturation/1
  consumption/1(consumption (liter)) -> [fuel_liter]
  Tice_ref/1 -> Product/1
  Oice/1 -> consumption/3(W_ice)
  Saturation/1 -> consumption/1(T_ice), Tice/1

== system HYV_EMR_IBC_Macro_2022a/Strategy block ==
  Ogear_estim : Inport
  Constant2 : Constant  Value=EMp.P_max
  Constant3 : Constant  Value=EMp.T_max
  MinMax1 : MinMax  Inputs=2
  Product3 : Product  Inputs=*/
  Saturation2 : Saturate  UpperLimit=Inf  LowerLimit=10.0
  T_lim : Outport  InitialOutput=0
  wires:
  Ogear_estim/1 -> Saturation2/1
  Constant2/1 -> Product3/1
  Saturation2/1 -> Product3/2
  Constant3/1 -> MinMax1/2
  Product3/1 -> MinMax1/1
  MinMax1/1 -> T_lim/1

== system HYV_EMR_IBC_Macro_2022a/Wheel ==
  Twh : Inport
  v_veh : Inport  Port=2
  Gain1 : Gain  Gain=1/MTp.R_wheel
  Gain2 : Gain  Gain=1/MTp.R_wheel
  Ftot : Outport  InitialOutput=0
  Owh : Outport  Port=2  InitialOutput=0
  wires:
  Gain1/1 -> Ftot/1
  Gain2/1 -> Owh/1
  v_veh/1 -> Gain2/1
  Twh/1 -> Gain1/1

== system HYV_EMR_IBC_Macro_2022a/BAT/Adaptation ==
  u_cell : Inport
  I_bat : Inport  Port=2
  Gain : Gain  Gain=BATp.ns
  Gain1 : Gain  Gain=1/BATp.np
  Memory : Memory
  u_bat : Outport  InitialOutput=0
  i_cell : Outport  Port=2  InitialOutput=0
  wires:
  Gain/1 -> u_bat/1
  I_bat/1 -> Gain1/1
  u_cell/1 -> Gain/1
  Gain1/1 -> Memory/1
  Memory/1 -> i_cell/1

== system HYV_EMR_IBC_Macro_2022a/BAT/Battery  cell resistance ==
  OCV : Inport
  icell : Inport  Port=2
  Gain : Gain  Gain=BATp.Rcell
  Subtract : Sum  Inputs=+-
  u_cell : Outport  InitialOutput=0
  I_cell : Outport  Port=2  InitialOutput=0
  wires:
  Subtract/1 -> u_cell/1
  icell/1 -> I_cell/1, Gain/1
  Gain/1 -> Subtract/2
  OCV/1 -> Subtract/1

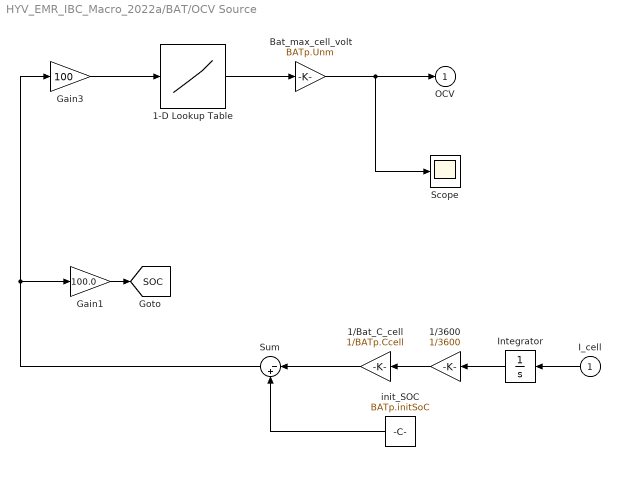
== system HYV_EMR_IBC_Macro_2022a/BAT/OCV Source ==
  "I_cell " : Inport
  1-D Lookup Table : Lookup_n-D  NumberOfTableDimensions=1  BreakpointsForDimension1=BATp.SoC  Table=BATp.OCV  InternalRulePriority=Speed  RndMeth=Simplest
  1/3600 : Gain  Gain=1/3600
  1/Bat_C_cell : Gain  Gain=1/BATp.Ccell
  Bat_max_cell_volt : Gain  Gain=BATp.Unm
  Gain1 : Gain  Gain=100.0
  Gain3 : Gain  Gain=100
  Integrator : Integrator
  Scope : Scope
  Sum : Sum  Inputs=|-+
  init_SOC : Constant  Value=BATp.initSoC
  OCV : Outport  InitialOutput=0
  tag scope: SOC=global
  wires:
  Sum/1 -> Gain1/1, Gain3/1
  1-D Lookup Table/1 -> Bat_max_cell_volt/1
  Gain3/1 -> 1-D Lookup Table/1
  Integrator/1 -> 1/3600/1
  init_SOC/1 -> Sum/2
  1/Bat_C_cell/1 -> Sum/1
  "I_cell "/1 -> Integrator/1
  1/3600/1 -> 1/Bat_C_cell/1
  Bat_max_cell_volt/1 -> Scope/1, OCV/1
  Gain1/1 -> [SOC]

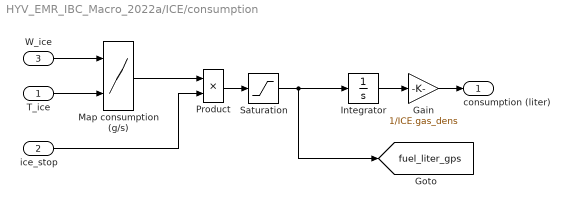
== system HYV_EMR_IBC_Macro_2022a/ICE/consumption ==
  T_ice : Inport
  ice_stop : Inport  Port=2
  W_ice : Inport  Port=3
  Gain : Gain  Gain=1/ICE.gas_dens  SaturateOnIntegerOverflow=on  OutDataTypeStr=Inherit: Same as input  ParamDataTypeStr=Inherit: Same as input
  Integrator : Integrator  LowerSaturationLimit=0
  Map consumption (g/s) : Lookup2D  RowIndex=ICE.Omega_def  ColumnIndex=ICE.Torque_def  Table=ICE.Fuel_consumption
  Product : Product  RndMeth=Zero
  Saturation : Saturate  UpperLimit=Inf  LowerLimit=0
  consumption (liter) : Outport  InitialOutput=0  VectorParamsAs1DForOutWhenUnconnected=off
  tag scope: fuel_liter_gps=global
  wires:
  ice_stop/1 -> Product/2
  Map consumption (g/s)/1 -> Product/1
  Product/1 -> Saturation/1
  Integrator/1 -> Gain/1
  W_ice/1 -> Map consumption (g/s)/1
  T_ice/1 -> Map consumption (g/s)/2
  Saturation/1 -> [fuel_liter_gps], Integrator/1
  Gain/1 -> consumption (liter)/1
